simulink model "PendulumSim"  (R2019a)
settings: Solver=VariableStepAuto  StartTime=0.0  StopTime=10.0  RelTol=1e-3
values from neighbouring files (symbols this model uses):
  b = 0.1    [PendulumTF.m]    (also in SelfBalanceScript.m)
  g = 9.8    [PIDtest.m]    (also in PendulumTF.m; SelfBalanceScript.m)
  I = 0.006    [PendulumTF.m]    (also in SelfBalanceScript.m)
  l = 12    [PIDtest.m]    (also in PendulumTF.m = 0.3; SelfBalanceAnim.m; SelfBalanceScript.m = 0.3)
  m = 0.2    [PendulumTF.m]    (also in SelfBalanceScript.m)
  M = feedback(G,H)    [PIDtest.m]    (also in PendulumTF.m = 0.5; SelfBalanceScript.m = 0.5)
settings Model: Creator=jornellq  LastModifiedBy=jornellq

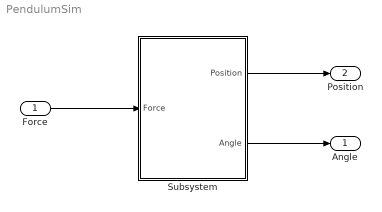
== system PendulumSim ==
  "Force " : Inport
  Subsystem : Subsystem
  "Angle " : Outport
  "Position " : Outport  Port=2
  wires:
  "Force "/1 -> Subsystem/1("Force ")
  Subsystem/1("Position ") -> "Position "/1
  Subsystem/2("Angle ") -> "Angle "/1

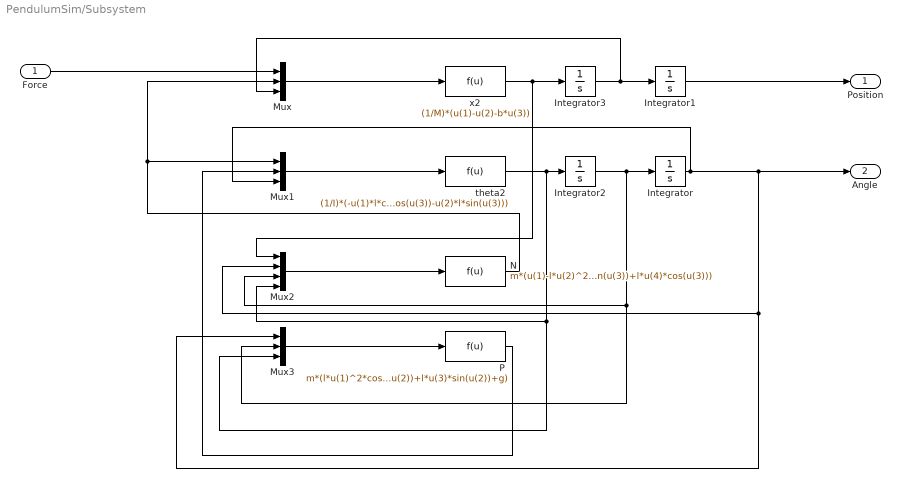
== system PendulumSim/Subsystem ==
  "Force " : Inport
  Integrator : Integrator  InitialCondition=pi  ContinuousStateAttributes='theta'
  Integrator1 : Integrator  ContinuousStateAttributes='x'
  Integrator2 : Integrator  ContinuousStateAttributes='theta1'
  Integrator3 : Integrator  ContinuousStateAttributes='x1'
  Mux : Mux  Inputs=3
  Mux1 : Mux  Inputs=3
  Mux2 : Mux
  Mux3 : Mux  Inputs=3
  N : Fcn  Expr=m*(u(1)-l*u(2)^2*sin(u(3))+l*u(4)*cos(u(3)))
  "P " : Fcn  Expr=m*(l*u(1)^2*cos(u(2))+l*u(3)*sin(u(2))+g)
  "theta2 " : Fcn  Expr=(1/I)*(-u(1)*l*cos(u(3))-u(2)*l*sin(u(3)))
  "x2 " : Fcn  Expr=(1/M)*(u(1)-u(2)-b*u(3))
  "Position " : Outport
  "Angle " : Outport  Port=2
  wires:
  "P "/1 -> Mux1/2
  Integrator3/1 -> Mux/3, Integrator1/1
  Mux/1 -> "x2 "/1
  N/1 -> Mux/2, Mux1/1
  Integrator2/1 -> Mux3/2, Mux2/3, Integrator/1
  Mux2/1 -> N/1
  Mux1/1 -> "theta2 "/1
  "Force "/1 -> Mux/1
  "x2 "/1 -> Mux2/1, Integrator3/1
  Integrator/1 -> Mux1/3, "Angle "/1, Mux3/1, Mux2/2
  "theta2 "/1 -> Mux3/3, Mux2/4, Integrator2/1
  Integrator1/1 -> "Position "/1
  Mux3/1 -> "P "/1
